simulink model "project_simulink"  (R2025a)
settings: Solver=VariableStepAuto  StartTime=0.0  StopTime=20  MaxStep=0.01  RelTol=1e-3
model workspace (MAT data in the model file):
  Diff_i = Simulink.Parameter
  Diff_i.Value = [1; 1; 1; 1]
  Diff_i.Complexity = 'real'
  Diff_i.Dimensions = [4 1]
  Diff_i.DataType = 'auto'
  Get_i = Simulink.Parameter
  Get_i.Value = [17; 16; 16; 17]
  Get_i.Complexity = 'real'
  Get_i.Dimensions = [4 1]
  Get_i.DataType = 'auto'
  Off_i = Simulink.Parameter
  Off_i.Value = [20; 20; 20; 20]
  Off_i.Complexity = 'real'
  Off_i.Dimensions = [4 1]
  Off_i.DataType = 'auto'
  On_i = Simulink.Parameter
  On_i.Value = [19; 19; 19; 19]
  On_i.Complexity = 'real'
  On_i.Dimensions = [4 1]
  On_i.DataType = 'auto'
  Room_Coefficients__A_ = Simulink.Parameter
  Room_Coefficients__A_.Value = [0  0.3  0.4  0.3; 0.3  0  0.5  0; 0.4  0.5  0  0.3; 0.3  0  0.3  0]
  Room_Coefficients__A_.Complexity = 'real'
  Room_Coefficients__A_.Dimensions = [4 4]
  Room_Coefficients__A_.DataType = 'auto'
  Thermal_Constant__Ci_ = Simulink.Parameter
  Thermal_Constant__Ci_.Value = [9; 7; 11; 7]
  Thermal_Constant__Ci_.Complexity = 'real'
  Thermal_Constant__Ci_.Dimensions = [4 1]
  Thermal_Constant__Ci_.DataType = 'auto'
  bi = Simulink.Parameter
  bi.Value = [0.3; 0.2; 0.5; 0.4]
  bi.Complexity = 'real'
  bi.Dimensions = [4 1]
  bi.DataType = 'auto'
  environment_temperature = Simulink.Parameter
  environment_temperature.Value = 6
  environment_temperature.Complexity = 'real'
  environment_temperature.Dimensions = [1 1]
  environment_temperature.DataType = 'auto'
  initial_temperature__x0_ = Simulink.Parameter
  initial_temperature__x0_.Value = [16.5; 16.5; 16.5; 16.5]
  initial_temperature__x0_.Complexity = 'real'
  initial_temperature__x0_.Dimensions = [4 1]
  initial_temperature__x0_.DataType = 'auto'
settings Model: Creator=Asus  LastModifiedBy=Asus
settings RTWCC: GPUComputeCapability=3.5

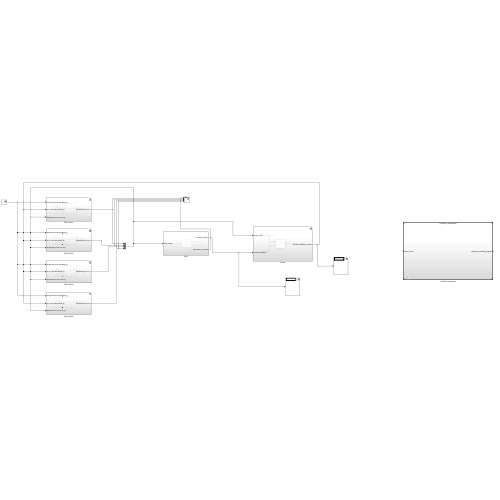
[thumbnail: Simulink's stored preview of the top-level diagram]
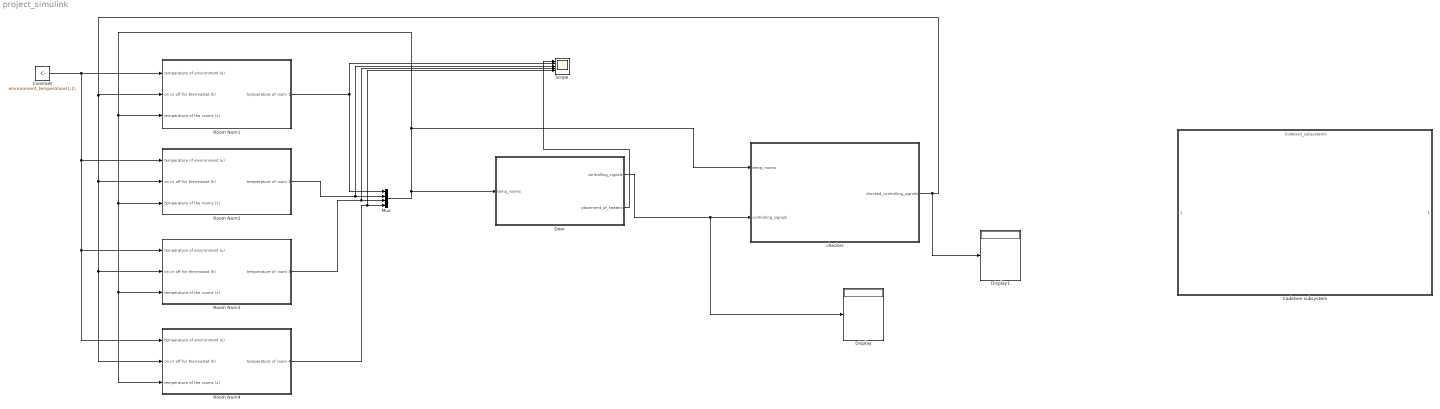
== system project_simulink ==
  CodeGen subsystem : ModelReference  ModelNameDialog=CodeGen_subsystem0  SimulationMode=Normal  ModelReferenceVersion=1.9
  Constant : Constant  Value=environment_temperature(1,1)
  Display : Display
  Display1 : Display
  Doer : Subsystem
  Mux : Mux
  Room Num1 : Subsystem
  Room Num2 : Subsystem
  Room Num3 : Subsystem
  Room Num4 : Subsystem
  Scope : Scope  NumInputPorts=5
      settings: ActiveDisplayYMinimum=11  ActiveDisplayYMaximum=35
  checker : Subsystem
  wires:
  Room Num1/1(temperature of room 1) -> Mux/1, Scope/2
  Room Num2/1(temperature of room 2) -> Scope/3, Mux/2
  Room Num3/1(temperature of room 3) -> Scope/4, Mux/3
  Room Num4/1(temperature of room 4) -> Scope/5, Mux/4
  Mux/1 -> Doer/1(temp_rooms), checker/1(temp_rooms), Room Num4/3(temperature of the rooms (x)), Room Num3/3(temperature of the rooms (x)), Room Num2/3(temperature of the rooms (x)), Room Num1/3(temperature of the rooms (x))
  Constant/1 -> Room Num4/1(temperature of environment (u)), Room Num3/1(temperature of environment (u)), Room Num2/1(temperature of environment (u)), Room Num1/1(temperature of environment (u))
  Doer/1(controlling_signals) -> Display/1, checker/2(controlling_signals)
  Doer/2(placement_of_heaters) -> Scope/1
  checker/1(checked_controlling_signals) -> Display1/1, Room Num4/2(on or off for thermostat (h)), Room Num3/2(on or off for thermostat (h)), Room Num2/2(on or off for thermostat (h)), Room Num1/2(on or off for thermostat (h))

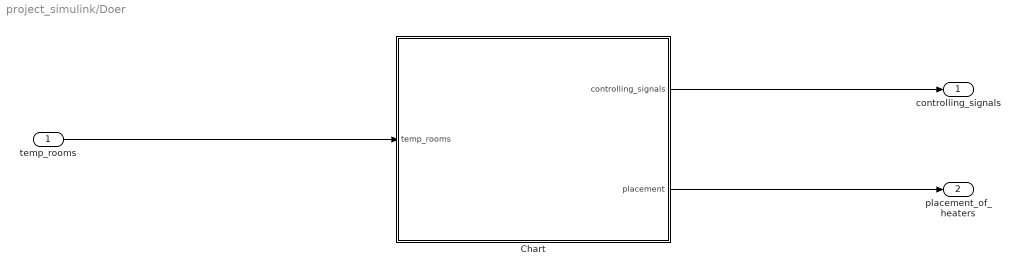
== system project_simulink/Doer ==
  temp_rooms : Inport
  Chart : Stateflow chart  TreatAsAtomicUnit=on
  controlling_signals : Outport
  placement_of_heaters : Outport  Port=2
  wires:
  temp_rooms/1 -> Chart/1(temp_rooms)
  Chart/1(controlling_signals) -> controlling_signals/1
  Chart/2(placement) -> placement_of_heaters/1

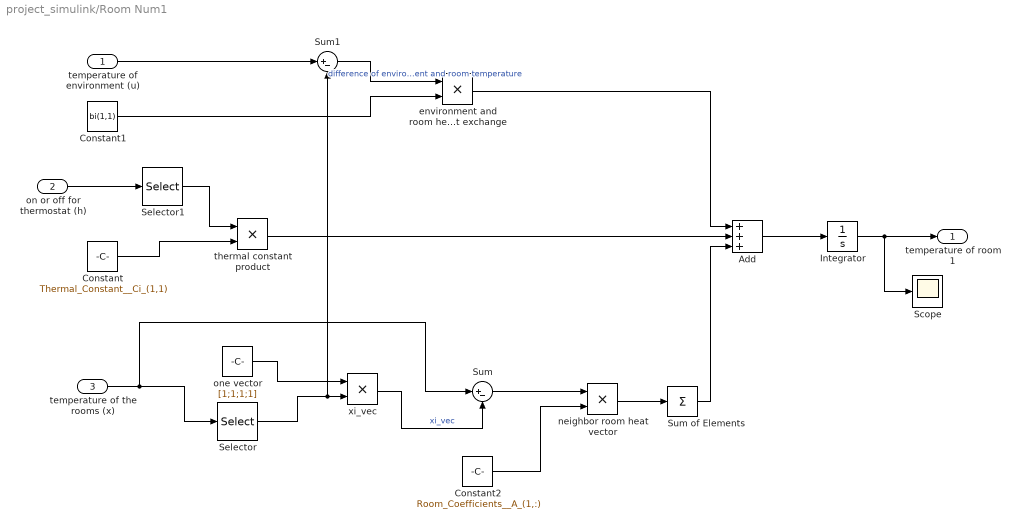
== system project_simulink/Room Num1 ==
  temperature of environment (u) : Inport
  on or off for thermostat (h) : Inport  Port=2
  temperature of the rooms (x) : Inport  Port=3  PortDimensions=4
  Add : Sum  Inputs=+++
  Constant : Constant  Value=Thermal_Constant__Ci_(1,1)
  Constant1 : Constant  Value=bi(1,1)
  Constant2 : Constant  Value=Room_Coefficients__A_(1,:)
  Integrator : Integrator  InitialCondition=initial_temperature__x0_(1,1)
  Scope : Scope
      settings: ActiveDisplayYMinimum=5.09005  ActiveDisplayYMaximum=17.76777
  Selector : Selector  InputPortWidth=4  IndexOptions=Index vector (dialog)  Indices=1  OutputSizes=1
  Selector1 : Selector  InputPortWidth=4  IndexOptions=Index vector (dialog)  Indices=1  OutputSizes=1
  Sum : Sum  Inputs=|+-
  Sum of Elements : Sum  Inputs=+
  Sum1 : Sum  Inputs=|+-
  environment and room heat exchange : Product
  neighbor room heat vector : Product
  one vector : Constant  Value=[1;1;1;1]
  thermal constant product : Product
  xi_vec : Product
  temperature of room 1 : Outport
  wires:
  Selector/1 -> Sum1/2, xi_vec/2
  one vector/1 -> xi_vec/1
  temperature of the rooms (x)/1 -> Sum/1, Selector/1
  xi_vec/1 -> Sum/2  "xi_vec"
  Sum/1 -> neighbor room heat vector/1
  Constant2/1 -> neighbor room heat vector/2
  neighbor room heat vector/1 -> Sum of Elements/1
  Constant/1 -> thermal constant product/2
  temperature of environment (u)/1 -> Sum1/1
  Constant1/1 -> environment and room heat exchange/2
  Sum1/1 -> environment and room heat exchange/1  "difference of environment and room temperature"
  environment and room heat exchange/1 -> Add/1
  thermal constant product/1 -> Add/2
  Sum of Elements/1 -> Add/3
  Add/1 -> Integrator/1
  Integrator/1 -> Scope/1, temperature of room 1/1
  on or off for thermostat (h)/1 -> Selector1/1
  Selector1/1 -> thermal constant product/1

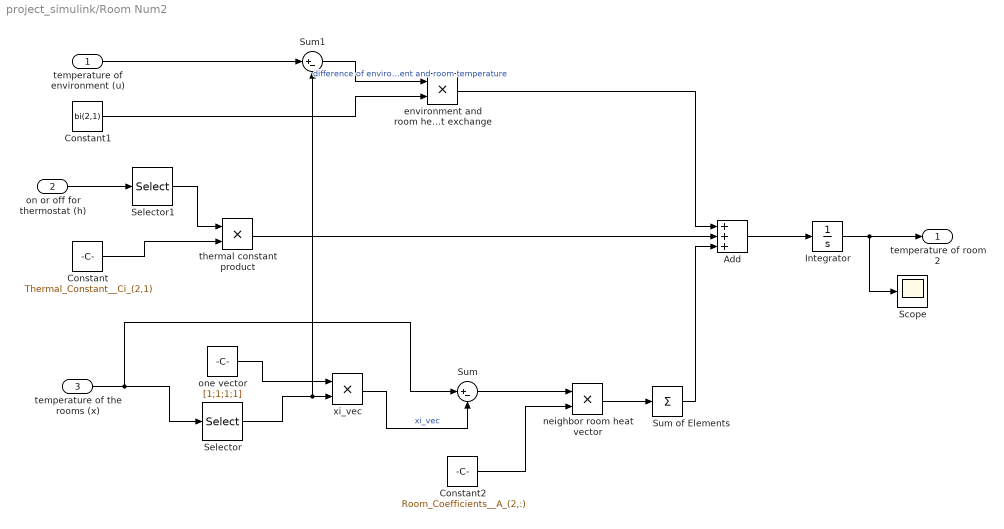
== system project_simulink/Room Num2 ==
  temperature of environment (u) : Inport
  on or off for thermostat (h) : Inport  Port=2
  temperature of the rooms (x) : Inport  Port=3  PortDimensions=4
  Add : Sum  Inputs=+++
  Constant : Constant  Value=Thermal_Constant__Ci_(2,1)
  Constant1 : Constant  Value=bi(2,1)
  Constant2 : Constant  Value=Room_Coefficients__A_(2,:)
  Integrator : Integrator  InitialCondition=initial_temperature__x0_(2,1)
  Scope : Scope
      settings: ActiveDisplayYMinimum=-1.19708  ActiveDisplayYMaximum=18.46634
  Selector : Selector  InputPortWidth=4  IndexOptions=Index vector (dialog)  Indices=2  OutputSizes=1
  Selector1 : Selector  InputPortWidth=4  IndexOptions=Index vector (dialog)  Indices=2  OutputSizes=1
  Sum : Sum  Inputs=|+-
  Sum of Elements : Sum  Inputs=+
  Sum1 : Sum  Inputs=|+-
  environment and room heat exchange : Product
  neighbor room heat vector : Product
  one vector : Constant  Value=[1;1;1;1]
  thermal constant product : Product
  xi_vec : Product
  temperature of room 2 : Outport
  wires:
  Sum/1 -> neighbor room heat vector/1
  temperature of environment (u)/1 -> Sum1/1
  Add/1 -> Integrator/1
  Sum1/1 -> environment and room heat exchange/1  "difference of environment and room temperature"
  Sum of Elements/1 -> Add/3
  Constant1/1 -> environment and room heat exchange/2
  Constant/1 -> thermal constant product/2
  environment and room heat exchange/1 -> Add/1
  Selector/1 -> Sum1/2, xi_vec/2
  temperature of the rooms (x)/1 -> Sum/1, Selector/1
  neighbor room heat vector/1 -> Sum of Elements/1
  xi_vec/1 -> Sum/2  "xi_vec"
  Constant2/1 -> neighbor room heat vector/2
  one vector/1 -> xi_vec/1
  thermal constant product/1 -> Add/2
  Integrator/1 -> Scope/1, temperature of room 2/1
  on or off for thermostat (h)/1 -> Selector1/1
  Selector1/1 -> thermal constant product/1

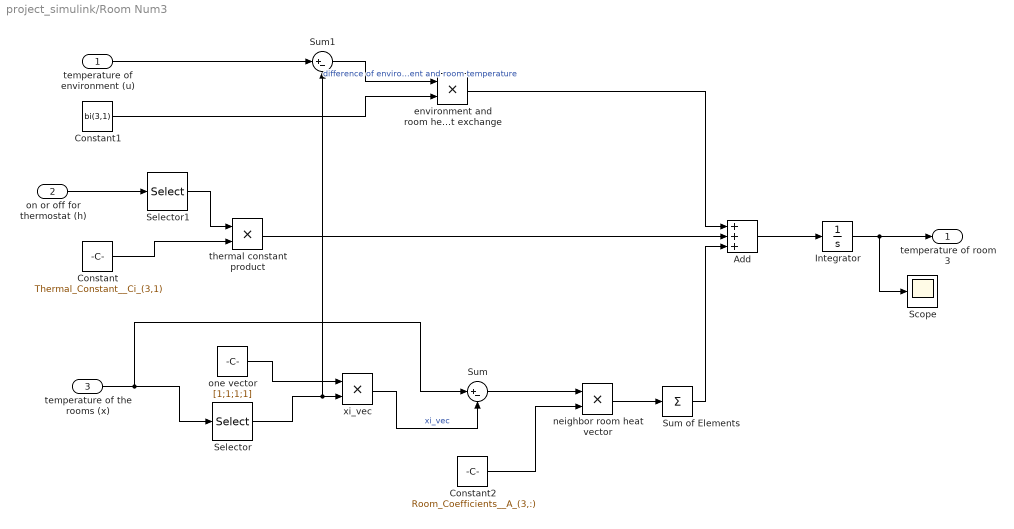
== system project_simulink/Room Num3 ==
  temperature of environment (u) : Inport
  on or off for thermostat (h) : Inport  Port=2
  temperature of the rooms (x) : Inport  Port=3  PortDimensions=4
  Add : Sum  Inputs=+++
  Constant : Constant  Value=Thermal_Constant__Ci_(3,1)
  Constant1 : Constant  Value=bi(3,1)
  Constant2 : Constant  Value=Room_Coefficients__A_(3,:)
  Integrator : Integrator  InitialCondition=initial_temperature__x0_(3,1)
  Scope : Scope
      settings: ActiveDisplayYMinimum=-1.19708  ActiveDisplayYMaximum=18.46634  DataLoggingVariableName=ScopeData2
  Selector : Selector  InputPortWidth=4  IndexOptions=Index vector (dialog)  Indices=3  OutputSizes=1
  Selector1 : Selector  InputPortWidth=4  IndexOptions=Index vector (dialog)  Indices=3  OutputSizes=1
  Sum : Sum  Inputs=|+-
  Sum of Elements : Sum  Inputs=+
  Sum1 : Sum  Inputs=|+-
  environment and room heat exchange : Product
  neighbor room heat vector : Product
  one vector : Constant  Value=[1;1;1;1]
  thermal constant product : Product
  xi_vec : Product
  temperature of room 3 : Outport
  wires:
  Sum/1 -> neighbor room heat vector/1
  temperature of environment (u)/1 -> Sum1/1
  Add/1 -> Integrator/1
  Sum1/1 -> environment and room heat exchange/1  "difference of environment and room temperature"
  Sum of Elements/1 -> Add/3
  Constant1/1 -> environment and room heat exchange/2
  Constant/1 -> thermal constant product/2
  on or off for thermostat (h)/1 -> Selector1/1
  environment and room heat exchange/1 -> Add/1
  Selector/1 -> Sum1/2, xi_vec/2
  temperature of the rooms (x)/1 -> Sum/1, Selector/1
  neighbor room heat vector/1 -> Sum of Elements/1
  xi_vec/1 -> Sum/2  "xi_vec"
  Constant2/1 -> neighbor room heat vector/2
  one vector/1 -> xi_vec/1
  thermal constant product/1 -> Add/2
  Integrator/1 -> Scope/1, temperature of room 3/1
  Selector1/1 -> thermal constant product/1

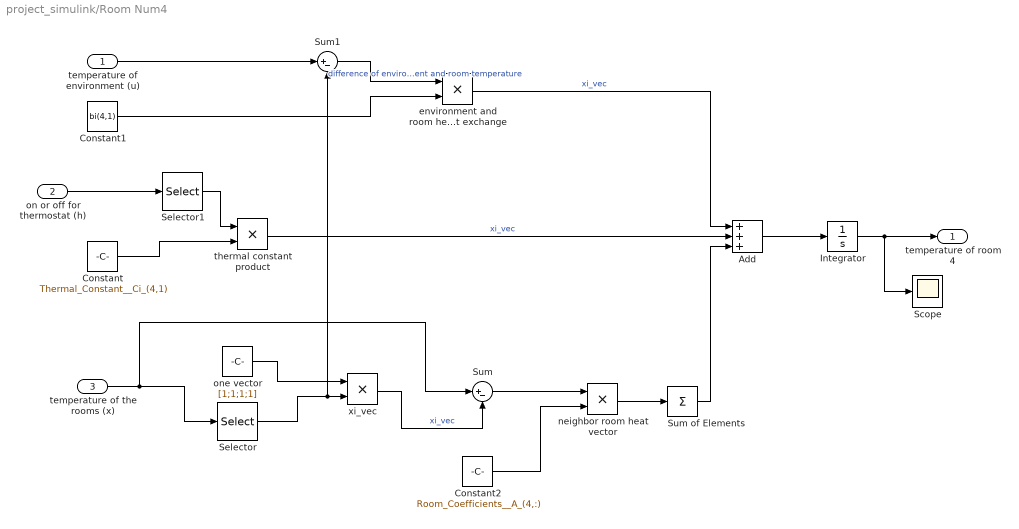
== system project_simulink/Room Num4 ==
  temperature of environment (u) : Inport
  on or off for thermostat (h) : Inport  Port=2
  temperature of the rooms (x) : Inport  Port=3  PortDimensions=4
  Add : Sum  Inputs=+++
  Constant : Constant  Value=Thermal_Constant__Ci_(4,1)
  Constant1 : Constant  Value=bi(4,1)
  Constant2 : Constant  Value=Room_Coefficients__A_(4,:)
  Integrator : Integrator  InitialCondition=initial_temperature__x0_(4,1)
  Scope : Scope
      settings: ActiveDisplayYMinimum=-1.19708  ActiveDisplayYMaximum=18.46634  DataLoggingVariableName=ScopeData3
  Selector : Selector  InputPortWidth=4  IndexOptions=Index vector (dialog)  Indices=4  OutputSizes=1
  Selector1 : Selector  InputPortWidth=4  IndexOptions=Index vector (dialog)  Indices=4  OutputSizes=1
  Sum : Sum  Inputs=|+-
  Sum of Elements : Sum  Inputs=+
  Sum1 : Sum  Inputs=|+-
  environment and room heat exchange : Product
  neighbor room heat vector : Product
  one vector : Constant  Value=[1;1;1;1]
  thermal constant product : Product
  xi_vec : Product
  temperature of room 4 : Outport
  wires:
  Sum/1 -> neighbor room heat vector/1
  temperature of environment (u)/1 -> Sum1/1
  Add/1 -> Integrator/1
  Sum1/1 -> environment and room heat exchange/1  "difference of environment and room temperature"
  Sum of Elements/1 -> Add/3
  Constant1/1 -> environment and room heat exchange/2
  Constant/1 -> thermal constant product/2
  environment and room heat exchange/1 -> Add/1  "xi_vec"
  Selector/1 -> Sum1/2, xi_vec/2
  temperature of the rooms (x)/1 -> Sum/1, Selector/1
  neighbor room heat vector/1 -> Sum of Elements/1
  xi_vec/1 -> Sum/2  "xi_vec"
  Constant2/1 -> neighbor room heat vector/2
  one vector/1 -> xi_vec/1
  thermal constant product/1 -> Add/2  "xi_vec"
  Integrator/1 -> Scope/1, temperature of room 4/1
  on or off for thermostat (h)/1 -> Selector1/1
  Selector1/1 -> thermal constant product/1

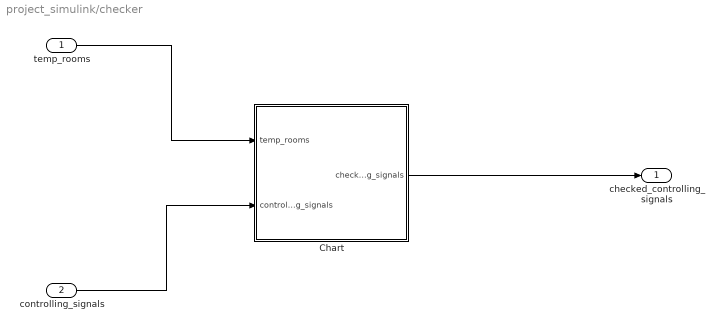
== system project_simulink/checker ==
  temp_rooms : Inport
  controlling_signals : Inport  Port=2
  Chart : Stateflow chart  TreatAsAtomicUnit=on
  checked_controlling_signals : Outport
  wires:
  temp_rooms/1 -> Chart/1(temp_rooms)
  controlling_signals/1 -> Chart/2(controlling_signals)
  Chart/1(checked_controlling_signals) -> checked_controlling_signals/1

== stateflow chart project_simulink/checker/Chart ==
  state safe
    during:
    checked_controlling_signals = controlling_signals
  state unsafe_sum
  (default) -> safe
  safe -> unsafe_sum : [sum(controlling_signals) > 2 || (controlling_signals(1) == 1 && temp_rooms(1) > Off_i(1)) || (controlling_signals(2) == 1 && temp_rooms(2) > Off_i(2)) || (controlling_signals(3) == 1 && temp_rooms(3) > Off_i(3)) || (controlling_signals(4) == 1 && temp_rooms(4) > Off_i(4))]{checked_controlling_signals(:) = 0}
  unsafe_sum -> safe : [~(sum(controlling_signals) > 2 || (controlling_signals(1) == 1 && temp_rooms(1) > Off_i(1)) || (controlling_signals(2) == 1 && temp_rooms(2) > Off_i(2)) || (controlling_signals(3) == 1 && temp_rooms(3) > Off_i(3)) || (controlling_signals(4) == 1 && temp_rooms(4) > Off_i(4)))]
  data: On_i parameter; Off_i parameter; temp_rooms input; controlling_signals input; checked_controlling_signals output =[0; 0; 0; 0]

== stateflow chart project_simulink/Doer/Chart ==
  state two_three
    during:
    placement = 23;
    if(temp_rooms(2) <= On_i(2))
    controlling_signals(2) = 1;
    end
    if(temp_rooms(3) <= On_i(3))
    controlling_signals(3) = 1;
    end
    if(temp_rooms(2) >= Off_i(2))
    controlling_signals(2) = 0;
    end
    if(temp_rooms(3) >= Off_i(3))
    controlling_signals(3) = 0;
    end
    exit:
    controlling_signals(:) = 0;
  state one_two
    during:
    placement = 12;
    if(temp_rooms(1) <= On_i(1))
    controlling_signals(1) = 1;
    end
    if(temp_rooms(2) <= On_i(2))
    controlling_signals(2) = 1;
    end
    if(temp_rooms(1) >= Off_i(1))
    controlling_signals(1) = 0;
    end
    if(temp_rooms(2) >= Off_i(2))
    controlling_signals(3) = 0;
    end
    exit:
    controlling_signals(:) = 0;
  state one_three
    during:
    placement = 13
    if(temp_rooms(1) <= On_i(1))
    controlling_signals(1) = 1;
    end
    if(temp_rooms(3) <= On_i(3))
    controlling_signals(3) = 1;
    end
    if(temp_rooms(1) >= Off_i(1))
    controlling_signals(1) = 0;
    end
    if(temp_rooms(3) >= Off_i(3))
    controlling_signals(3) = 0;
    end
    exit:
    controlling_signals(:) = 0;
  state one_four
    during:
    placement = 14;
    if(temp_rooms(1) <= On_i(1))
    controlling_signals(1) = 1;
    end
    if(temp_rooms(4) <= On_i(4))
    controlling_signals(4) = 1;
    end
    if(temp_rooms(1) >= Off_i(1))
    controlling_signals(1) = 0;
    end
    if(temp_rooms(4) >= Off_i(4))
    controlling_signals(4) = 0;
    end
    exit:
    controlling_signals(:) = 0;
  state two_four
    during:
    placement = 24;
    if(temp_rooms(2) <= On_i(2))
    controlling_signals(2) = 1;
    end
    if(temp_rooms(4) <= On_i(4))
    controlling_signals(4) = 1;
    end
    if(temp_rooms(2) >= Off_i(2))
    controlling_signals(2) = 0;
    end
    if(temp_rooms(4) >= Off_i(4))
    controlling_signals(4) = 0;
    end
    exit:
    controlling_signals(:) = 0;
  state three_four
    during:
    placement = 34;
    if(temp_rooms(3) <= On_i(3))
    controlling_signals(3) = 1;
    end
    if(temp_rooms(4) <= On_i(4))
    controlling_signals(4) = 1;
    end
    if(temp_rooms(3) >= Off_i(3))
    controlling_signals(3) = 0;
    end
    if(temp_rooms(4) >= Off_i(4))
    controlling_signals(4) = 0;
    end
    exit:
    controlling_signals(:) = 0;
  one_three -> two_three [order 3] : [temp_rooms(1) - temp_rooms(2) >= Diff_i(2) && temp_rooms(2) <= Get_i(2)]
  two_three -> one_three [order 3] : [temp_rooms(2) - temp_rooms(1) >= Diff_i(1) && temp_rooms(1) <= Get_i(1)]
  one_three -> one_four [order 2] : [temp_rooms(3) - temp_rooms(4) >= Diff_i(4) && temp_rooms(4) <= Get_i(4)]
  (default) -> two_three
  one_two -> one_three [order 3] : [temp_rooms(2) - temp_rooms(3) >= Diff_i(3) && temp_rooms(3) <= Get_i(3)]
  two_three -> one_two [order 1] : [temp_rooms(3) - temp_rooms(1) >= Diff_i(1) && temp_rooms(1) <= Get_i(1)]
  one_three -> one_two [order 1] : [temp_rooms(3) - temp_rooms(2) >= Diff_i(2) && temp_rooms(2) <= Get_i(2)]
  one_two -> two_three [order 1] : [temp_rooms(1) - temp_rooms(3) >= Diff_i(3) && temp_rooms(3) <= Get_i(3)]
  one_two -> one_four [order 4] : [temp_rooms(2) - temp_rooms(4) >= Diff_i(4) && temp_rooms(4) <= Get_i(4)]
  three_four -> two_three [order 3] : [temp_rooms(4) - temp_rooms(2) >= Diff_i(2) && temp_rooms(2) <= Get_i(2)]
  two_four -> two_three [order 4] : [temp_rooms(4) - temp_rooms(3) >= Diff_i(3) && temp_rooms(3) <= Get_i(3)]
  two_three -> three_four [order 4] : [temp_rooms(2) - temp_rooms(4) >= Diff_i(4) && temp_rooms(4) <= Get_i(4)]
  two_three -> two_four [order 2] : [temp_rooms(3) - temp_rooms(4) >= Diff_i(4) && temp_rooms(4) <= Get_i(4)]
  one_four -> one_two [order 3] : [temp_rooms(4) - temp_rooms(2) >= Diff_i(2) && temp_rooms(2) <= Get_i(2)]
  one_four -> one_three [order 4] : [temp_rooms(4) - temp_rooms(3) >= Diff_i(3) && temp_rooms(3) <= Get_i(3)]
  one_two -> two_four [order 2] : [temp_rooms(1) - temp_rooms(4) >= Diff_i(4) && temp_rooms(4) <= Get_i(4)]
  two_four -> one_two [order 3] : [temp_rooms(4) - temp_rooms(1) >= Diff_i(1) && temp_rooms(1) <= Get_i(1)]
  one_three -> three_four [order 4] : [temp_rooms(3) - temp_rooms(1) >= Diff_i(1) && temp_rooms(1) <= Get_i(1)]
  three_four -> one_three [order 4] : [temp_rooms(4) - temp_rooms(1) >= Diff_i(1) && temp_rooms(1) <= Get_i(1)]
  one_four -> two_four [order 1] : [temp_rooms(1) - temp_rooms(2) >= Diff_i(2) && temp_rooms(2) <= Get_i(2)]
  two_four -> three_four [order 2] : [temp_rooms(2) - temp_rooms(3) >= Diff_i(3) && temp_rooms(3) <= Get_i(3)]
  three_four -> two_four [order 1] : [temp_rooms(3) - temp_rooms(2) >= Diff_i(2) && temp_rooms(2) <= Get_i(2)]
  two_four -> one_four [order 1] : [temp_rooms(2) - temp_rooms(1) >= Diff_i(1) && temp_rooms(1) <= Get_i(1)]
  three_four -> one_four [order 2] : [temp_rooms(3) - temp_rooms(1) >= Diff_i(1) && temp_rooms(1) <= Get_i(1)]
  one_four -> three_four [order 2] : [temp_rooms(1) - temp_rooms(3) >= Diff_i(3) && temp_rooms(3) <= Get_i(3)]
  data: On_i parameter; Off_i parameter; Get_i parameter; Diff_i parameter; temp_rooms input size=[4 1]; controlling_signals output =[0; 0; 0; 0]; placement output
